simulink model "str_speed"  (Simulink 7.4)
settings: Solver=FixedStepDiscrete  StartTime=0.0  StopTime=20  FixedStep=0.005  RelTol=1e-3
settings Model: Creator=NGUYEN VINH HAO  LastModifiedBy=Admin
settings OptimizationCC: OptimizeModelRefInitCode=on  LifeSpan=1
settings RTWCC: SystemTargetFile=ert.tlc  GenCodeOnly=on  GenerateMakefile=off  TemplateMakefile=ert_default_tmf  Description=Real-Time Workshop Embedded Coder  ProcessScript=ert_make_rtw_hook
settings CodeAppCC: IgnoreCustomStorageClasses=off
settings ERTTargetCC: MultiwordLength=2048  GenerateSampleERTMain=on  ERTCustomFileTemplate=example_file_process.tlc  ConvertIfToSwitch=off

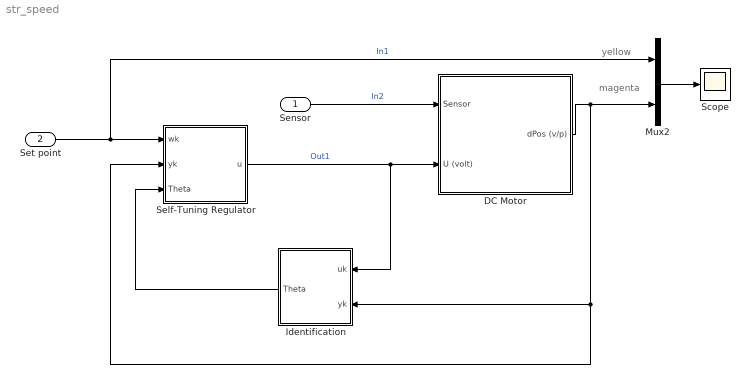
== system str_speed ==
  note: yellow
  note: magenta
  Sensor : Inport  PortDimensions=1  OutDataType=sfix(16)  OutScaling=2^0
  Set point : Inport  Port=2  PortDimensions=1  OutDataType=sfix(16)  OutScaling=2^0
  DC Motor : Subsystem
  Identification : Subsystem
  Mux2 : Mux  Inputs=2
  Scope : Scope
      settings: YMin=1999.78  YMax=2000.03
  Self-Tuning Regulator : Subsystem
  wires:
  Sensor/1 -> DC Motor/1(Sensor)  "In2"
  Self-Tuning Regulator/1(u) -> DC Motor/2(U (volt)), Identification/1(uk)  "Out1"
  Mux2/1 -> Scope/1
  Identification/1(Theta) -> Self-Tuning Regulator/3(Theta)
  Set point/1 -> Mux2/1, Self-Tuning Regulator/1(wk)  "In1"
  DC Motor/1(dPos (v/p)) -> Mux2/2, Identification/2(yk), Self-Tuning Regulator/2(yk)

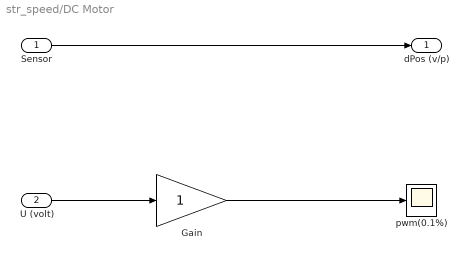
== system str_speed/DC Motor ==
  Sensor : Inport  PortDimensions=1  OutDataType=sfix(16)  OutScaling=2^0
  U (volt) : Inport  Port=2  PortDimensions=1  OutDataType=sfix(16)  OutScaling=2^0
  Gain : Gain  ParameterDataType=sfix(16)  ParameterScaling=2^0  OutDataType=sfix(16)  OutScaling=2^0  ParamDataTypeStr=Inherit: Same as input
  pwm(0.1%) : Scope
      settings: YMin=-1100  YMax=1100  SaveName=ScopeData3  DataFormat=Array
  dPos (v/p) : Outport  PortDimensions=1  OutDataType=sfix(16)  OutScaling=2^0
  wires:
  U (volt)/1 -> Gain/1
  Sensor/1 -> dPos (v/p)/1
  Gain/1 -> pwm(0.1%)/1

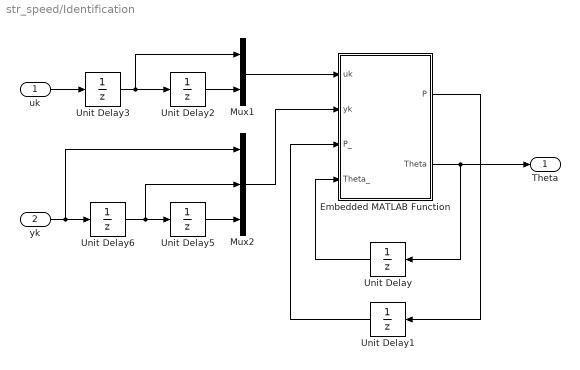
== system str_speed/Identification ==
  uk : Inport  PortDimensions=1  OutDataType=fixdt(1, 16)  OutScaling=2^0
  yk : Inport  Port=2  PortDimensions=1  OutDataType=fixdt(1, 16)  OutScaling=2^0
  Embedded MATLAB Function : Stateflow chart
  Mux1 : Mux  Inputs=2
  Mux2 : Mux  Inputs=3
  Unit Delay : UnitDelay  X0=[-1; 0.1; 0.1; 1]  SampleTime=-1
  Unit Delay1 : UnitDelay  X0=1e5*eye(4)  SampleTime=-1
  Unit Delay{2..3,5..6} (4 alike) : UnitDelay  SampleTime=-1
  Theta : Outport  PortDimensions=4  OutDataType=fixdt(1, 16)  OutScaling=2^0
  wires:
  Unit Delay/1 -> Embedded MATLAB Function/4(Theta_)
  Embedded MATLAB Function/2(Theta) -> Unit Delay/1, Theta/1
  Unit Delay1/1 -> Embedded MATLAB Function/3(P_)
  Embedded MATLAB Function/1(P) -> Unit Delay1/1
  Mux1/1 -> Embedded MATLAB Function/1(uk)
  Unit Delay6/1 -> Mux2/2, Unit Delay5/1
  Unit Delay5/1 -> Mux2/3
  Mux2/1 -> Embedded MATLAB Function/2(yk)
  Unit Delay2/1 -> Mux1/2
  Unit Delay3/1 -> Unit Delay2/1, Mux1/1
  uk/1 -> Unit Delay3/1
  yk/1 -> Unit Delay6/1, Mux2/1

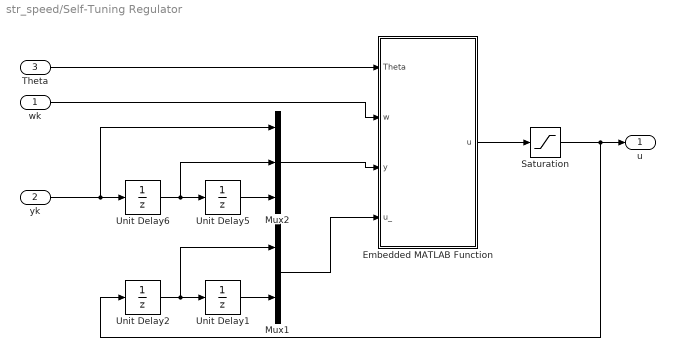
== system str_speed/Self-Tuning Regulator ==
  wk : Inport  PortDimensions=1  OutDataType=fixdt(1, 16)  OutScaling=2^0
  yk : Inport  Port=2  PortDimensions=1  OutDataType=fixdt(1, 16)  OutScaling=2^0
  Theta : Inport  Port=3  PortDimensions=4  OutDataType=sfix(16)  OutScaling=2^0
  Embedded MATLAB Function : Stateflow chart
  Mux1 : Mux  Inputs=2
  Mux2 : Mux  Inputs=3
  Saturation : Saturate  UpperLimit=10  LowerLimit=-10  OutDataType=fixdt(1, 16)  OutScaling=2^0
  Unit Delay{1..2,5..6} (4 alike) : UnitDelay  SampleTime=-1
  u : Outport  PortDimensions=1  OutDataType=fixdt(1, 16)  OutScaling=2^0
  wires:
  wk/1 -> Embedded MATLAB Function/2(w)
  Mux2/1 -> Embedded MATLAB Function/3(y)
  Theta/1 -> Embedded MATLAB Function/1(Theta)
  yk/1 -> Mux2/1, Unit Delay6/1
  Mux1/1 -> Embedded MATLAB Function/4(u_)
  Unit Delay1/1 -> Mux1/2
  Unit Delay2/1 -> Mux1/1, Unit Delay1/1
  Embedded MATLAB Function/1(u) -> Saturation/1
  Unit Delay5/1 -> Mux2/3
  Unit Delay6/1 -> Unit Delay5/1, Mux2/2
  Saturation/1 -> Unit Delay2/1, u/1

== matlab function Identification/Embedded MATLAB Function ==
  settings: fimath=|
      | fimath(...
      | 'RoundMode', 'floor',...
      | 'OverflowMode', 'wrap',...
      | 'ProductMode', 'KeepLSB', 'ProductWordLength', 32,...
      | 'SumMode', 'KeepLSB', 'SumWordLength', 32,...
      | 'CastBeforeSum', false)
  data: P output double; uk input double; yk input double; P_ input double; Theta_ input double; Theta output double
function [P,Theta] = Uocluong(uk,yk,P_,Theta_)

lamda = 0.95;
PHI = [-yk(2); -yk(3); uk(1); uk(2)];
e = yk(1) - PHI'*Theta_;
L = P_*PHI/(lamda+PHI'*P_*PHI);
P = 1/lamda*(P_-(P_*PHI)*(PHI'*P_)/(lamda+PHI'*P_*PHI));
Theta = Theta_ + L*e;

== matlab function Self-Tuning Regulator/Embedded MATLAB Function ==
  settings: fimath=|
      | fimath(...
      | 'RoundMode', 'floor',...
      | 'OverflowMode', 'wrap',...
      | 'ProductMode', 'KeepLSB', 'ProductWordLength', 32,...
      | 'SumMode', 'KeepLSB', 'SumWordLength', 32,...
      | 'CastBeforeSum', false)
  data: Theta input double; u output double; w input double; y input double; u_ input double
function u = STR_pp2(Theta,w,y,u_)

% Cai dat cap cuc (mien roi rac) mong muon
beta = 0.1;
alpha = 0.6;
% Gan lai cho de su dung
a1 = Theta(1);
a2 = Theta(2);
b1 = Theta(3);
b2 = Theta(4);
% Sinh vien tham khao huong dan Muc 2.4.2 de viet bo sung code
x1 = -4*alpha + 1 - a1;
x2 = 6*alpha^2 + beta^2 + a1 - a2;
x3 = 2*alpha*(2*alpha^2+beta^2) - a2;
x4 = alpha^2*(alpha^2+beta^2);

r1 = (b1+b2)*(a1*b1*b2-a2*b1^2-b2^2);
r2 = a1*b2*(b1*(x2-x3+x4)-b2*x1);
r3 = a2*b1*(b2*x1-b1*(x2-x3+x4));
r4 = (b1+b2)*(b1*x4+b2*(x3-x4));
r5 = b1*(b1^2*x4+b1*b2*x3+b2^2*x2)-b2^3*x1;
r6 = b1^2*(a2*x3+a1*x4-a2*x4);
r7 = b2*(b1*(a1*x4+a2*x2-x4)-b2*(a2*x1+x4));

r0 = (x1+x2-x3+x4)/(b1+b2);
p1 = (r5 - r1)/r1;
p2 = -(r5/r1);
q0 = r0 - (r2+r3+r4)/r1;
q1 = (r2+r3+r4-r6-r7)/r1;
q2 = (r6+r7)/r1;

% Luat dieu khien
u = r0*w - q0*y(1) - q1*y(2) - q2*y(3) - p1*u_(1) - p2*u_(2);
